simulink library "slctrlextras"  (Simulink 7.6)
settings: Solver=ode45  SolverMode=SingleTasking  StartTime=0.0  StopTime=10.0  RelTol=1e-3
undefined symbols (not defined in the file or in its folder): SnapshotTimes
libraries: simulink x4, slctrlblks x1
settings Model: Creator=jglass  LastModifiedBy=astother

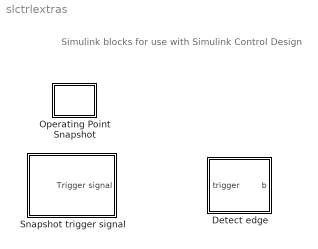
== system slctrlextras ==
  note: Simulink blocks for use with Simulink Control Design
  Detect edge : Subsystem  mask{TriggerType=rising, ZeroCross=on}
      mask prompts: TriggerType "Trigger type:"; ZeroCross "Enable zero crossing detection"
      mask help: Implemented trigger detection block.
      mask init:
      | slctrlblkdlgs.configTriggerBlk(gcbh)
      mask StyleString: popup(rising|falling),checkbox
      mask Display: disp('Rising')
  Operating Point Snapshot : Subsystem  mask(Time Operating Condition Snapshot){SnapshotTimes=[1 2]}
      mask prompts: SnapshotTimes "Operating point snapshot times:"
      mask help: Generate linear models in the base workspace at specific times.
      mask Help: This block calls LINMOD or DLINMOD to create a linear model for the system when the simulation clock reaches the time specified by the LinearizationTime parameter.  No trimming is performed.  The linear model is stored in the base workspace as a structure, along with information about the operating point at which the snapshot was taken.  Multiple snapshots are appended to form an array of structures.
      mask Display: disp(['T=' mat2str(SnapshotTimes)])
  Snapshot trigger signal : Subsystem

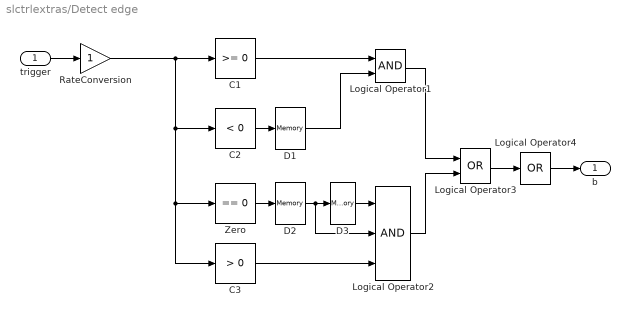
== system slctrlextras/Detect edge ==
  trigger : Inport
  C1 : simulink/Logic and Bit Operations/Compare To Zero  SystemSampleTime=-1  relop=>=  LogicOutDataTypeMode=uint8
  C2 : simulink/Logic and Bit Operations/Compare To Zero  SystemSampleTime=-1  relop=<  LogicOutDataTypeMode=uint8
  C3 : simulink/Logic and Bit Operations/Compare To Zero  SystemSampleTime=-1  relop=>  LogicOutDataTypeMode=uint8
  D1 : Memory
  D2 : Memory
  D3 : Memory
  Logical Operator1 : Logic  AllPortsSameDT=off  OutDataTypeMode=boolean  LogicDataType=fixdt(0, 8)  OutDataTypeStr=boolean
  Logical Operator2 : Logic  Inputs=3  AllPortsSameDT=off  OutDataTypeMode=boolean  LogicDataType=fixdt(0, 8)  OutDataTypeStr=boolean
  Logical Operator3 : Logic  Operator=OR  AllPortsSameDT=off  OutDataTypeMode=boolean  LogicDataType=fixdt(0, 8)  OutDataTypeStr=boolean
  Logical Operator4 : Logic  Operator=OR  Inputs=1  AllPortsSameDT=off  OutDataTypeMode=boolean  LogicDataType=fixdt(0, 8)  OutDataTypeStr=boolean
  RateConversion : Gain  ParameterDataType=fixdt(1, 16)  ParameterScaling=2^0  OutDataType=fixdt(1, 16)  OutScaling=2^0
  Zero : simulink/Logic and Bit Operations/Compare To Zero  SystemSampleTime=-1  relop===  LogicOutDataTypeMode=uint8
  b : Outport
  wires:
  trigger/1 -> RateConversion/1
  C1/1 -> Logical Operator1/1
  C2/1 -> D1/1
  Zero/1 -> D2/1
  Logical Operator1/1 -> Logical Operator3/1
  Logical Operator2/1 -> Logical Operator3/2
  Logical Operator3/1 -> Logical Operator4/1
  D1/1 -> Logical Operator1/2
  D2/1 -> D3/1, Logical Operator2/2
  D3/1 -> Logical Operator2/1
  C3/1 -> Logical Operator2/3
  Logical Operator4/1 -> b/1
  RateConversion/1 -> C1/1, C2/1, C3/1, Zero/1

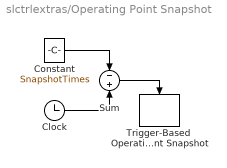
== system slctrlextras/Operating Point Snapshot ==
  Clock : Clock
      settings: Decimation=10
  Constant : Constant  Value=SnapshotTimes  OutDataType=sfix(16)  OutScaling=2^0
  Sum : Sum  Inputs=-+  OutDataType=sfix(16)  OutScaling=2^0  SaturateOnIntegerOverflow=on  InputSameDT=on  OutDataTypeStr=Inherit: Same as first input
  Trigger-Based  Operating Point Snapshot : slctrlblks/Trigger-Based  Operating Point Snapshot  TriggerType=rising
  wires:
  Sum/1 -> Trigger-Based  Operating Point Snapshot/Trigger
  Constant/1 -> Sum/1
  Clock/1 -> Sum/2

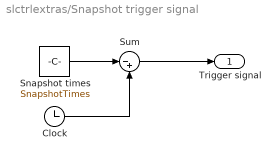
== system slctrlextras/Snapshot trigger signal ==
  Clock : Clock
      settings: Decimation=10
  Snapshot times : Constant  Value=SnapshotTimes  OutDataType=fixdt(1, 16)  OutScaling=2^0
  Sum : Sum  Inputs=|-+  OutDataType=fixdt(1, 16)  OutScaling=2^0
  Trigger signal : Outport
  wires:
  Sum/1 -> Trigger signal/1
  Snapshot times/1 -> Sum/1
  Clock/1 -> Sum/2
